simulink model "LFTBasico"  (R2019a)
settings: Solver=VariableStepAuto  StartTime=0.0  StopTime=10.0  RelTol=1e-3
libraries: cstblocks x2, simulink_extras x1
settings Model: Creator=marcos.pesante  LastModifiedBy=marcos.pesante

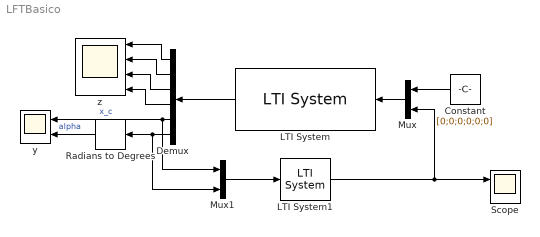
== system LFTBasico ==
  Constant : Constant  Value=[0;0;0;0;0;0]
  Demux : Demux  Outputs=6
  LTI System : cstblocks/LTI System  sys=unc_sys.NominalValue  IC=[]
  LTI System1 : cstblocks/LTI System  sys=K  IC=[]
  Mux : Mux  Inputs=2
  Mux1 : Mux  Inputs=2
  Radians to Degrees : simulink_extras/Transformations/Radians to Degrees
  Scope : Scope  NumInputPorts=2
  y : Scope  NumInputPorts=2
  z : Scope  NumInputPorts=4
  wires:
  LTI System1/1 -> Mux/2, Scope/1
  Constant/1 -> Mux/1
  Mux/1 -> LTI System/1
  LTI System/1 -> Demux/1
  Demux/1 -> z/1
  Demux/2 -> z/2
  Demux/3 -> z/3
  Demux/4 -> z/4
  Demux/5 -> y/1, Mux1/1  "x_c"
  Demux/6 -> Mux1/2, Radians to Degrees/1
  Mux1/1 -> LTI System1/1
  Radians to Degrees/1 -> y/2  "alpha"
